simulink library "Thermal_Node"  (Simulink 8.2)
settings: Solver=ode45  StartTime=0.0  StopTime=10.0  RelTol=1e-3
settings Model: Creator=drhf  LastModifiedBy=drhf

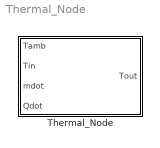
== system Thermal_Node ==
  Thermal_Node : Subsystem  mask(Thermal Capacity){UA=1, mcp=10*4182, cp_approx=4182, Tini=20}
      mask prompts: UA "Loss coefficient of node in W/K"; mcp "Thermal capacity of the node (mcp) in J/K"; cp_approx "Heat capacity of entering massflow in J/kg/K (approximate value)"; Tini "Initial temperature in °C"
      mask help:
      | Basic one node model of a thermal mass using the differential equation:
      | mcp * dT/dt = UA_loss*(Tamb-T) + mdot*cp_in*(Tin-T) + Qdot
      | Qdot: additional thermal power added to node
      | mdot: entering massflow
      | Tin: temperature of entering massflow
      mask Help: web(fullfile(path_carnot('help'),'Thermal_Capacity.html'),'-helpbrowser')
      mask Display: plot(-20,0,120,100,[10,70,70,10,10],[10,10,70,70,10],[70,90,90,30,10],[10,30,90,90,70],[90,70],[90,70],[50,30],[60,60],[40,40],[30,60])

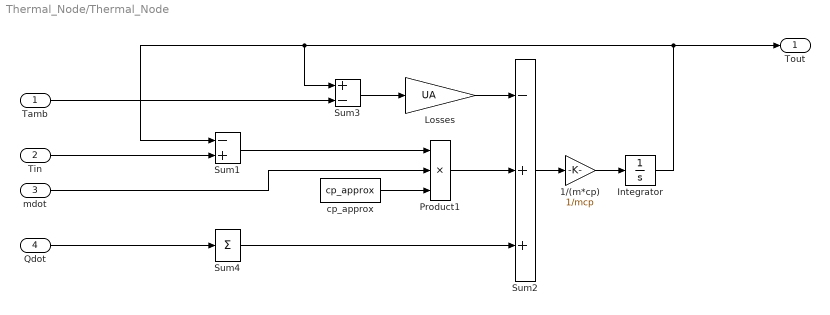
== system Thermal_Node/Thermal_Node ==
  Tamb : Inport
  Tin : Inport  Port=2
  mdot : Inport  Port=3
  Qdot : Inport  Port=4
  1/(m*cp) : Gain  Gain=1/mcp  SaturateOnIntegerOverflow=on  OutDataTypeStr=Inherit: Same as input  ParamDataTypeStr=Inherit: Same as input
  Integrator : Integrator  InitialCondition=Tini
  Losses : Gain  Gain=UA  SaturateOnIntegerOverflow=on  OutDataTypeStr=Inherit: Same as input  ParamDataTypeStr=Inherit: Same as input
  Product1 : Product  Inputs=3  SaturateOnIntegerOverflow=on  InputSameDT=on  OutDataTypeStr=Inherit: Same as first input
  Sum1 : Sum  Inputs=-+  SaturateOnIntegerOverflow=on  InputSameDT=on  OutDataTypeStr=Inherit: Same as first input
  Sum2 : Sum  Inputs=-++  SaturateOnIntegerOverflow=on  InputSameDT=on  OutDataTypeStr=Inherit: Same as first input
  Sum3 : Sum  Inputs=+-  SaturateOnIntegerOverflow=on  InputSameDT=on  OutDataTypeStr=Inherit: Same as first input
  Sum4 : Sum  Inputs=1  SaturateOnIntegerOverflow=on  InputSameDT=on  OutDataTypeStr=Inherit: Same as first input
  cp_approx : Constant  Value=cp_approx
  Tout : Outport
  wires:
  Sum4/1 -> Sum2/3
  Sum1/1 -> Product1/1
  1/(m*cp)/1 -> Integrator/1
  cp_approx/1 -> Product1/3
  Sum3/1 -> Losses/1
  Losses/1 -> Sum2/1
  Tamb/1 -> Sum3/2
  Sum2/1 -> 1/(m*cp)/1
  Product1/1 -> Sum2/2
  Integrator/1 -> Tout/1, Sum3/1, Sum1/1
  Tin/1 -> Sum1/2
  mdot/1 -> Product1/2
  Qdot/1 -> Sum4/1
